simulink model "Demo_STM"  (R2020a)
settings: Solver=VariableStepAuto  StartTime=0.0  StopTime=inf  RelTol=1e-3
settings Model: Creator=steal  LastModifiedBy=steal

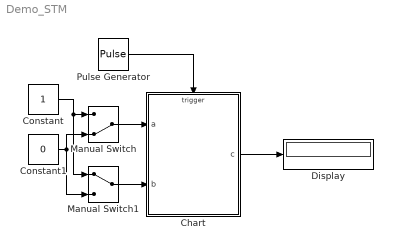
== system Demo_STM ==
  Chart : Stateflow chart  TreatAsAtomicUnit=on
  Constant : Constant
  Constant1 : Constant  Value=0
  Display : Display
  Manual Switch : ManualSwitch  CurrentSetting=0
  Manual Switch1 : ManualSwitch
  Pulse Generator : DiscretePulseGenerator  Period=10  PulseWidth=5  SampleTime=1e-3
  wires:
  Constant/1 -> Manual Switch1/1, Manual Switch/1
  Manual Switch1/1 -> Chart/2(b)
  Manual Switch/1 -> Chart/1(a)
  Constant1/1 -> Manual Switch/2, Manual Switch1/2
  Chart/1(c) -> Display/1
  Pulse Generator/1 -> Chart/Trigger

== stateflow chart Demo_STM/Chart ==
  state State1
    entry: c=1;
  state State2
    during: c = a + 5;
  state State3
    entry: c=0;
  state State4
  (default) -> State1
  State4 -> State1 : [hasChanged(b)]
  State1 -> State2 : [a==1]
  State2 -> State3 : [b == 1]
  State3 -> State4 : [after(5,sec)]{c=5}
  data: a input; b input; c output
  events: event input RISING_EDGE_EVENT
